simulink model "Experiment3_time_model"  (R2012b)
settings: Solver=ode1  StartTime=0.0  StopTime=simulink_time  FixedStep=step_size  RelTol=1e-3
values from neighbouring files (symbols this model uses):
  exp_model = 1    [model_ref.mat]
  exp_model_input = 1    [model_input.mat]
undefined symbols (not defined in the file or in its folder): K, Plant_K, Plant_T1, Plant_T2, simulink_start_time, T1, T2
settings Model: Creator=Administrator  LastModifiedBy=Administrator

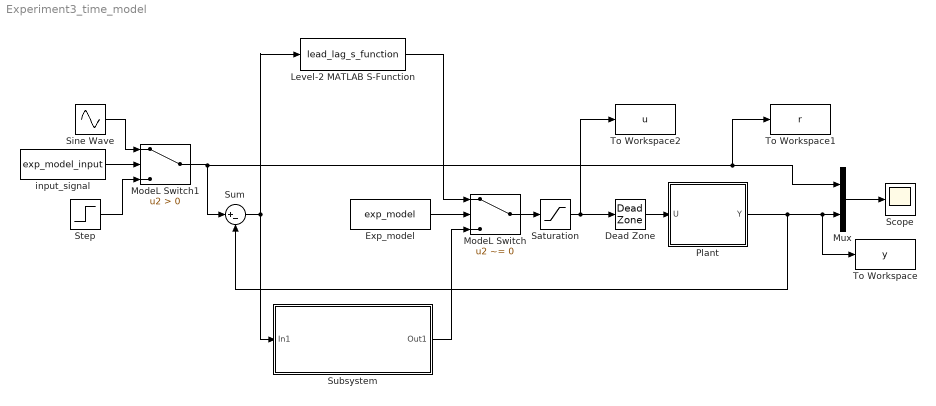
== system Experiment3_time_model ==
  Dead Zone : DeadZone  LowerValue=-2  UpperValue=2  SaturateOnIntegerOverflow=on
  Exp_model : Constant  Value=exp_model
  Level-2 MATLAB S-Function : M-S-Function  FunctionName=lead_lag_s_function  Parameters=lead_lag_params
  ModeL Switch : Switch  Criteria=u2 ~= 0
  ModeL Switch1 : Switch  Criteria=u2 > Threshold
  Mux : Mux  Inputs=2
  Plant : Subsystem
  Saturation : Saturate  UpperLimit=19.2  LowerLimit=-19.2
  Scope : Scope
      settings: TimeRange=5
  Sine Wave : Sin  Amplitude=20  Frequency=2*pi*5  SampleTime=0
  Step : Step  Time=simulink_start_time  After=60  SampleTime=0
  Subsystem : Subsystem
  Sum : Sum  Inputs=|+-
  To Workspace : ToWorkspace  VariableName=y  SampleTime=-1
  To Workspace1 : ToWorkspace  VariableName=r  SampleTime=-1
  To Workspace2 : ToWorkspace  VariableName=u  SampleTime=-1
  input_signal : Constant  Value=exp_model_input
  wires:
  ModeL Switch1/1 -> Sum/1, To Workspace1/1, Mux/1
  Mux/1 -> Scope/1
  ModeL Switch/1 -> Saturation/1
  Exp_model/1 -> ModeL Switch/2
  Step/1 -> ModeL Switch1/3
  input_signal/1 -> ModeL Switch1/2
  Sine Wave/1 -> ModeL Switch1/1
  Saturation/1 -> Dead Zone/1, To Workspace2/1
  Dead Zone/1 -> Plant/1(U)
  Plant/1(Y) -> Sum/2, To Workspace/1, Mux/2
  Sum/1 -> Subsystem/1(In1), Level-2 MATLAB S-Function/1
  Subsystem/1(Out1) -> ModeL Switch/3
  Level-2 MATLAB S-Function/1 -> ModeL Switch/1

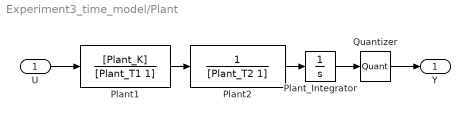
== system Experiment3_time_model/Plant ==
  U : Inport
  Plant1 : TransferFcn  Numerator=[Plant_K]  Denominator=[Plant_T1 1]
  Plant2 : TransferFcn  Denominator=[Plant_T2 1]
  Plant_Integrator : Integrator
  Quantizer : Quantizer  QuantizationInterval=0.005
  Y : Outport
  wires:
  U/1 -> Plant1/1
  Quantizer/1 -> Y/1
  Plant1/1 -> Plant2/1
  Plant_Integrator/1 -> Quantizer/1
  Plant2/1 -> Plant_Integrator/1

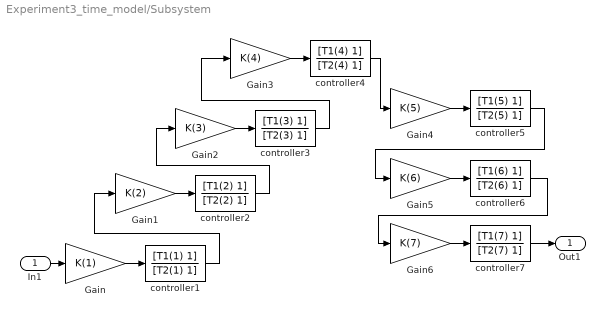
== system Experiment3_time_model/Subsystem ==
  In1 : Inport
  Gain : Gain  Gain=K(1)
  Gain1 : Gain  Gain=K(2)
  Gain2 : Gain  Gain=K(3)
  Gain3 : Gain  Gain=K(4)
  Gain4 : Gain  Gain=K(5)
  Gain5 : Gain  Gain=K(6)
  Gain6 : Gain  Gain=K(7)
  controller1 : TransferFcn  Numerator=[T1(1) 1]  Denominator=[T2(1) 1]
  controller2 : TransferFcn  Numerator=[T1(2) 1]  Denominator=[T2(2) 1]
  controller3 : TransferFcn  Numerator=[T1(3) 1]  Denominator=[T2(3) 1]
  controller4 : TransferFcn  Numerator=[T1(4) 1]  Denominator=[T2(4) 1]
  controller5 : TransferFcn  Numerator=[T1(5) 1]  Denominator=[T2(5) 1]
  controller6 : TransferFcn  Numerator=[T1(6) 1]  Denominator=[T2(6) 1]
  controller7 : TransferFcn  Numerator=[T1(7) 1]  Denominator=[T2(7) 1]
  Out1 : Outport
  wires:
  Gain/1 -> controller1/1
  In1/1 -> Gain/1
  Gain1/1 -> controller2/1
  controller1/1 -> Gain1/1
  Gain2/1 -> controller3/1
  controller2/1 -> Gain2/1
  Gain3/1 -> controller4/1
  controller3/1 -> Gain3/1
  Gain4/1 -> controller5/1
  controller4/1 -> Gain4/1
  Gain5/1 -> controller6/1
  controller5/1 -> Gain5/1
  Gain6/1 -> controller7/1
  controller6/1 -> Gain6/1
  controller7/1 -> Out1/1
